simulink model "SensorFaultInj"  (R2013a)
settings: Solver=FixedStepDiscrete  SolverMode=SingleTasking  StartTime=0.0  StopTime=SimLength  FixedStep=SampleTime  RelTol=1e-3
values from neighbouring files (symbols this model uses):
  GlobalSeed = 10    [start_framework07.m]
  SampleTime = 0.01    [start_framework07.m]
  SimLength = 40    [start_framework07.m]
undefined symbols (not defined in the file or in its folder): DiscIntNeverNeededParam
libraries: dspswit3 x48, simulink x32
(part 9 of 9)

== system SensorFaultInj/FIM_Muster1/Parser Modul/parameter parser/Enabled Subsystem/param_fcn id 9/parser_fcn param id 2 ==
  input : Inport
  ex_sfun_paramfcn : S-Function  FunctionName=ex_sfun_paramfcn  EnableBusSupport=off  mask(Legacy Function){SFunctionSpec=double y1 = param_fcn(single u1, single u2, single u3), ShowSpec=on}
      mask prompts: ShowSpec "Display function specification"
      mask help:
      | This block allows you to call the legacy functions specified by the following Legacy Code Tool definition:
      | def.SFunctionName = 'ex_sfun_paramfcn';
      | def.OutputFcnSpec = 'double y1 = param_fcn(single u1, single u2, single u3)';
      | def.HeaderFiles = {'param_fcn.hpp'};
      | def.SourceFiles = {'param_fcn.cpp'};
      | def.Options.language = 'C++';
      mask Help: <p>This block was generated automatically by the Legacy Code Tool. For detailed help on this tool, call<a href="matlab:legacy_code('help')"> legacy_code('help')</a>.</p>
      mask Callback ShowSpec:
      | if strcmp(get_param(gcbh, 'ShowSpec'), 'on')
      |   set_param(gcbh, 'MaskDisplay', sprintf('fprintf(''%s'');', get_param(gcbh, 'SFunctionSpec')));
      | else
      |   set_param(gcbh, 'MaskDisplay', sprintf('fprintf(''%s'');', get_param(gcbh, 'FunctionName')));
      | end
      mask Display: fprintf('double y1 = param_fcn(single u1, single u2, single u3)');
  "fault_id " : Constant  Value=9  OutDataTypeStr=single
  "param_id " : Constant  Value=0  OutDataTypeStr=single
  output : Outport
  wires:
  "fault_id "/1 -> ex_sfun_paramfcn/1
  "param_id "/1 -> ex_sfun_paramfcn/2
  ex_sfun_paramfcn/1 -> output/1
  input/1 -> ex_sfun_paramfcn/3

== system SensorFaultInj/FIM_Muster1/Parser Modul/parameter parser/Enabled Subsystem/param_fcn id 9/parser_fcn param id 3 ==
  input : Inport
  ex_sfun_paramfcn : S-Function  FunctionName=ex_sfun_paramfcn  EnableBusSupport=off  mask(Legacy Function){SFunctionSpec=double y1 = param_fcn(single u1, single u2, single u3), ShowSpec=on}
      mask prompts: ShowSpec "Display function specification"
      mask help:
      | This block allows you to call the legacy functions specified by the following Legacy Code Tool definition:
      | def.SFunctionName = 'ex_sfun_paramfcn';
      | def.OutputFcnSpec = 'double y1 = param_fcn(single u1, single u2, single u3)';
      | def.HeaderFiles = {'param_fcn.hpp'};
      | def.SourceFiles = {'param_fcn.cpp'};
      | def.Options.language = 'C++';
      mask Help: <p>This block was generated automatically by the Legacy Code Tool. For detailed help on this tool, call<a href="matlab:legacy_code('help')"> legacy_code('help')</a>.</p>
      mask Callback ShowSpec:
      | if strcmp(get_param(gcbh, 'ShowSpec'), 'on')
      |   set_param(gcbh, 'MaskDisplay', sprintf('fprintf(''%s'');', get_param(gcbh, 'SFunctionSpec')));
      | else
      |   set_param(gcbh, 'MaskDisplay', sprintf('fprintf(''%s'');', get_param(gcbh, 'FunctionName')));
      | end
      mask Display: fprintf('double y1 = param_fcn(single u1, single u2, single u3)');
  "fault_id " : Constant  Value=9  OutDataTypeStr=single
  "param_id " : Constant  OutDataTypeStr=single
  output : Outport
  wires:
  "fault_id "/1 -> ex_sfun_paramfcn/1
  "param_id "/1 -> ex_sfun_paramfcn/2
  ex_sfun_paramfcn/1 -> output/1
  input/1 -> ex_sfun_paramfcn/3

== system SensorFaultInj/FIM_Muster2/Parser Modul/parameter parser/Enabled Subsystem/param_fcn id 0/parser_fcn param id 2 ==
  input : Inport
  ex_sfun_paramfcn : S-Function  FunctionName=ex_sfun_paramfcn  EnableBusSupport=off  mask(Legacy Function){SFunctionSpec=double y1 = param_fcn(single u1, single u2, single u3), ShowSpec=on}
      mask prompts: ShowSpec "Display function specification"
      mask help:
      | This block allows you to call the legacy functions specified by the following Legacy Code Tool definition:
      | def.SFunctionName = 'ex_sfun_paramfcn';
      | def.OutputFcnSpec = 'double y1 = param_fcn(single u1, single u2, single u3)';
      | def.HeaderFiles = {'param_fcn.hpp'};
      | def.SourceFiles = {'param_fcn.cpp'};
      | def.Options.language = 'C++';
      mask Help: <p>This block was generated automatically by the Legacy Code Tool. For detailed help on this tool, call<a href="matlab:legacy_code('help')"> legacy_code('help')</a>.</p>
      mask Callback ShowSpec:
      | if strcmp(get_param(gcbh, 'ShowSpec'), 'on')
      |   set_param(gcbh, 'MaskDisplay', sprintf('fprintf(''%s'');', get_param(gcbh, 'SFunctionSpec')));
      | else
      |   set_param(gcbh, 'MaskDisplay', sprintf('fprintf(''%s'');', get_param(gcbh, 'FunctionName')));
      | end
      mask Display: fprintf('double y1 = param_fcn(single u1, single u2, single u3)');
  "fault_id " : Constant  Value=0  OutDataTypeStr=single
  "param_id " : Constant  Value=0  OutDataTypeStr=single
  output : Outport
  wires:
  "fault_id "/1 -> ex_sfun_paramfcn/1
  "param_id "/1 -> ex_sfun_paramfcn/2
  ex_sfun_paramfcn/1 -> output/1
  input/1 -> ex_sfun_paramfcn/3

== system SensorFaultInj/FIM_Muster2/Parser Modul/parameter parser/Enabled Subsystem/param_fcn id 1/parser_fcn param id 2 ==
  input : Inport
  ex_sfun_paramfcn : S-Function  FunctionName=ex_sfun_paramfcn  EnableBusSupport=off  mask(Legacy Function){SFunctionSpec=double y1 = param_fcn(single u1, single u2, single u3), ShowSpec=on}
      mask prompts: ShowSpec "Display function specification"
      mask help:
      | This block allows you to call the legacy functions specified by the following Legacy Code Tool definition:
      | def.SFunctionName = 'ex_sfun_paramfcn';
      | def.OutputFcnSpec = 'double y1 = param_fcn(single u1, single u2, single u3)';
      | def.HeaderFiles = {'param_fcn.hpp'};
      | def.SourceFiles = {'param_fcn.cpp'};
      | def.Options.language = 'C++';
      mask Help: <p>This block was generated automatically by the Legacy Code Tool. For detailed help on this tool, call<a href="matlab:legacy_code('help')"> legacy_code('help')</a>.</p>
      mask Callback ShowSpec:
      | if strcmp(get_param(gcbh, 'ShowSpec'), 'on')
      |   set_param(gcbh, 'MaskDisplay', sprintf('fprintf(''%s'');', get_param(gcbh, 'SFunctionSpec')));
      | else
      |   set_param(gcbh, 'MaskDisplay', sprintf('fprintf(''%s'');', get_param(gcbh, 'FunctionName')));
      | end
      mask Display: fprintf('double y1 = param_fcn(single u1, single u2, single u3)');
  "fault_id " : Constant  OutDataTypeStr=single
  "param_id " : Constant  Value=0  OutDataTypeStr=single
  output : Outport
  wires:
  "fault_id "/1 -> ex_sfun_paramfcn/1
  "param_id "/1 -> ex_sfun_paramfcn/2
  ex_sfun_paramfcn/1 -> output/1
  input/1 -> ex_sfun_paramfcn/3

== system SensorFaultInj/FIM_Muster2/Parser Modul/parameter parser/Enabled Subsystem/param_fcn id 10/parser_fcn param id 0 ==
  input : Inport
  ex_sfun_paramfcn : S-Function  FunctionName=ex_sfun_paramfcn  EnableBusSupport=off  mask(Legacy Function){SFunctionSpec=double y1 = param_fcn(single u1, single u2, single u3), ShowSpec=on}
      mask prompts: ShowSpec "Display function specification"
      mask help:
      | This block allows you to call the legacy functions specified by the following Legacy Code Tool definition:
      | def.SFunctionName = 'ex_sfun_paramfcn';
      | def.OutputFcnSpec = 'double y1 = param_fcn(single u1, single u2, single u3)';
      | def.HeaderFiles = {'param_fcn.hpp'};
      | def.SourceFiles = {'param_fcn.cpp'};
      | def.Options.language = 'C++';
      mask Help: <p>This block was generated automatically by the Legacy Code Tool. For detailed help on this tool, call<a href="matlab:legacy_code('help')"> legacy_code('help')</a>.</p>
      mask Callback ShowSpec:
      | if strcmp(get_param(gcbh, 'ShowSpec'), 'on')
      |   set_param(gcbh, 'MaskDisplay', sprintf('fprintf(''%s'');', get_param(gcbh, 'SFunctionSpec')));
      | else
      |   set_param(gcbh, 'MaskDisplay', sprintf('fprintf(''%s'');', get_param(gcbh, 'FunctionName')));
      | end
      mask Display: fprintf('double y1 = param_fcn(single u1, single u2, single u3)');
  "fault_id " : Constant  Value=10  OutDataTypeStr=single
  "param_id " : Constant  Value=0  OutDataTypeStr=single
  output : Outport
  wires:
  "fault_id "/1 -> ex_sfun_paramfcn/1
  "param_id "/1 -> ex_sfun_paramfcn/2
  ex_sfun_paramfcn/1 -> output/1
  input/1 -> ex_sfun_paramfcn/3

== system SensorFaultInj/FIM_Muster2/Parser Modul/parameter parser/Enabled Subsystem/param_fcn id 10/parser_fcn param id 1 ==
  input : Inport
  ex_sfun_paramfcn : S-Function  FunctionName=ex_sfun_paramfcn  EnableBusSupport=off  mask(Legacy Function){SFunctionSpec=double y1 = param_fcn(single u1, single u2, single u3), ShowSpec=on}
      mask prompts: ShowSpec "Display function specification"
      mask help:
      | This block allows you to call the legacy functions specified by the following Legacy Code Tool definition:
      | def.SFunctionName = 'ex_sfun_paramfcn';
      | def.OutputFcnSpec = 'double y1 = param_fcn(single u1, single u2, single u3)';
      | def.HeaderFiles = {'param_fcn.hpp'};
      | def.SourceFiles = {'param_fcn.cpp'};
      | def.Options.language = 'C++';
      mask Help: <p>This block was generated automatically by the Legacy Code Tool. For detailed help on this tool, call<a href="matlab:legacy_code('help')"> legacy_code('help')</a>.</p>
      mask Callback ShowSpec:
      | if strcmp(get_param(gcbh, 'ShowSpec'), 'on')
      |   set_param(gcbh, 'MaskDisplay', sprintf('fprintf(''%s'');', get_param(gcbh, 'SFunctionSpec')));
      | else
      |   set_param(gcbh, 'MaskDisplay', sprintf('fprintf(''%s'');', get_param(gcbh, 'FunctionName')));
      | end
      mask Display: fprintf('double y1 = param_fcn(single u1, single u2, single u3)');
  "fault_id " : Constant  Value=10  OutDataTypeStr=single
  "param_id " : Constant  OutDataTypeStr=single
  output : Outport
  wires:
  "fault_id "/1 -> ex_sfun_paramfcn/1
  "param_id "/1 -> ex_sfun_paramfcn/2
  ex_sfun_paramfcn/1 -> output/1
  input/1 -> ex_sfun_paramfcn/3

== system SensorFaultInj/FIM_Muster2/Parser Modul/parameter parser/Enabled Subsystem/param_fcn id 11/parser_fcn param id 2 ==
  input : Inport
  ex_sfun_paramfcn : S-Function  FunctionName=ex_sfun_paramfcn  EnableBusSupport=off  mask(Legacy Function){SFunctionSpec=double y1 = param_fcn(single u1, single u2, single u3), ShowSpec=on}
      mask prompts: ShowSpec "Display function specification"
      mask help:
      | This block allows you to call the legacy functions specified by the following Legacy Code Tool definition:
      | def.SFunctionName = 'ex_sfun_paramfcn';
      | def.OutputFcnSpec = 'double y1 = param_fcn(single u1, single u2, single u3)';
      | def.HeaderFiles = {'param_fcn.hpp'};
      | def.SourceFiles = {'param_fcn.cpp'};
      | def.Options.language = 'C++';
      mask Help: <p>This block was generated automatically by the Legacy Code Tool. For detailed help on this tool, call<a href="matlab:legacy_code('help')"> legacy_code('help')</a>.</p>
      mask Callback ShowSpec:
      | if strcmp(get_param(gcbh, 'ShowSpec'), 'on')
      |   set_param(gcbh, 'MaskDisplay', sprintf('fprintf(''%s'');', get_param(gcbh, 'SFunctionSpec')));
      | else
      |   set_param(gcbh, 'MaskDisplay', sprintf('fprintf(''%s'');', get_param(gcbh, 'FunctionName')));
      | end
      mask Display: fprintf('double y1 = param_fcn(single u1, single u2, single u3)');
  "fault_id " : Constant  Value=11  OutDataTypeStr=single
  "param_id " : Constant  Value=0  OutDataTypeStr=single
  output : Outport
  wires:
  "fault_id "/1 -> ex_sfun_paramfcn/1
  "param_id "/1 -> ex_sfun_paramfcn/2
  ex_sfun_paramfcn/1 -> output/1
  input/1 -> ex_sfun_paramfcn/3

== system SensorFaultInj/FIM_Muster2/Parser Modul/parameter parser/Enabled Subsystem/param_fcn id 12/parser_fcn param id 2 ==
  input : Inport
  ex_sfun_paramfcn : S-Function  FunctionName=ex_sfun_paramfcn  EnableBusSupport=off  mask(Legacy Function){SFunctionSpec=double y1 = param_fcn(single u1, single u2, single u3), ShowSpec=on}
      mask prompts: ShowSpec "Display function specification"
      mask help:
      | This block allows you to call the legacy functions specified by the following Legacy Code Tool definition:
      | def.SFunctionName = 'ex_sfun_paramfcn';
      | def.OutputFcnSpec = 'double y1 = param_fcn(single u1, single u2, single u3)';
      | def.HeaderFiles = {'param_fcn.hpp'};
      | def.SourceFiles = {'param_fcn.cpp'};
      | def.Options.language = 'C++';
      mask Help: <p>This block was generated automatically by the Legacy Code Tool. For detailed help on this tool, call<a href="matlab:legacy_code('help')"> legacy_code('help')</a>.</p>
      mask Callback ShowSpec:
      | if strcmp(get_param(gcbh, 'ShowSpec'), 'on')
      |   set_param(gcbh, 'MaskDisplay', sprintf('fprintf(''%s'');', get_param(gcbh, 'SFunctionSpec')));
      | else
      |   set_param(gcbh, 'MaskDisplay', sprintf('fprintf(''%s'');', get_param(gcbh, 'FunctionName')));
      | end
      mask Display: fprintf('double y1 = param_fcn(single u1, single u2, single u3)');
  "fault_id " : Constant  Value=12  OutDataTypeStr=single
  "param_id " : Constant  Value=0  OutDataTypeStr=single
  output : Outport
  wires:
  "fault_id "/1 -> ex_sfun_paramfcn/1
  "param_id "/1 -> ex_sfun_paramfcn/2
  ex_sfun_paramfcn/1 -> output/1
  input/1 -> ex_sfun_paramfcn/3

== system SensorFaultInj/FIM_Muster2/Parser Modul/parameter parser/Enabled Subsystem/param_fcn id 2/parser_fcn param id 3 ==
  input : Inport
  ex_sfun_paramfcn : S-Function  FunctionName=ex_sfun_paramfcn  EnableBusSupport=off  mask(Legacy Function){SFunctionSpec=double y1 = param_fcn(single u1, single u2, single u3), ShowSpec=on}
      mask prompts: ShowSpec "Display function specification"
      mask help:
      | This block allows you to call the legacy functions specified by the following Legacy Code Tool definition:
      | def.SFunctionName = 'ex_sfun_paramfcn';
      | def.OutputFcnSpec = 'double y1 = param_fcn(single u1, single u2, single u3)';
      | def.HeaderFiles = {'param_fcn.hpp'};
      | def.SourceFiles = {'param_fcn.cpp'};
      | def.Options.language = 'C++';
      mask Help: <p>This block was generated automatically by the Legacy Code Tool. For detailed help on this tool, call<a href="matlab:legacy_code('help')"> legacy_code('help')</a>.</p>
      mask Callback ShowSpec:
      | if strcmp(get_param(gcbh, 'ShowSpec'), 'on')
      |   set_param(gcbh, 'MaskDisplay', sprintf('fprintf(''%s'');', get_param(gcbh, 'SFunctionSpec')));
      | else
      |   set_param(gcbh, 'MaskDisplay', sprintf('fprintf(''%s'');', get_param(gcbh, 'FunctionName')));
      | end
      mask Display: fprintf('double y1 = param_fcn(single u1, single u2, single u3)');
  "fault_id " : Constant  Value=2  OutDataTypeStr=single
  "param_id " : Constant  Value=0  OutDataTypeStr=single
  output : Outport
  wires:
  "fault_id "/1 -> ex_sfun_paramfcn/1
  "param_id "/1 -> ex_sfun_paramfcn/2
  ex_sfun_paramfcn/1 -> output/1
  input/1 -> ex_sfun_paramfcn/3

== system SensorFaultInj/FIM_Muster2/Parser Modul/parameter parser/Enabled Subsystem/param_fcn id 3/parser_fcn param id 2 ==
  input : Inport
  ex_sfun_paramfcn : S-Function  FunctionName=ex_sfun_paramfcn  EnableBusSupport=off  mask(Legacy Function){SFunctionSpec=double y1 = param_fcn(single u1, single u2, single u3), ShowSpec=on}
      mask prompts: ShowSpec "Display function specification"
      mask help:
      | This block allows you to call the legacy functions specified by the following Legacy Code Tool definition:
      | def.SFunctionName = 'ex_sfun_paramfcn';
      | def.OutputFcnSpec = 'double y1 = param_fcn(single u1, single u2, single u3)';
      | def.HeaderFiles = {'param_fcn.hpp'};
      | def.SourceFiles = {'param_fcn.cpp'};
      | def.Options.language = 'C++';
      mask Help: <p>This block was generated automatically by the Legacy Code Tool. For detailed help on this tool, call<a href="matlab:legacy_code('help')"> legacy_code('help')</a>.</p>
      mask Callback ShowSpec:
      | if strcmp(get_param(gcbh, 'ShowSpec'), 'on')
      |   set_param(gcbh, 'MaskDisplay', sprintf('fprintf(''%s'');', get_param(gcbh, 'SFunctionSpec')));
      | else
      |   set_param(gcbh, 'MaskDisplay', sprintf('fprintf(''%s'');', get_param(gcbh, 'FunctionName')));
      | end
      mask Display: fprintf('double y1 = param_fcn(single u1, single u2, single u3)');
  "fault_id " : Constant  Value=3  OutDataTypeStr=single
  "param_id " : Constant  Value=0  OutDataTypeStr=single
  output : Outport
  wires:
  "fault_id "/1 -> ex_sfun_paramfcn/1
  "param_id "/1 -> ex_sfun_paramfcn/2
  ex_sfun_paramfcn/1 -> output/1
  input/1 -> ex_sfun_paramfcn/3

== system SensorFaultInj/FIM_Muster2/Parser Modul/parameter parser/Enabled Subsystem/param_fcn id 4/parser_fcn param id 2 ==
  input : Inport
  ex_sfun_paramfcn : S-Function  FunctionName=ex_sfun_paramfcn  EnableBusSupport=off  mask(Legacy Function){SFunctionSpec=double y1 = param_fcn(single u1, single u2, single u3), ShowSpec=on}
      mask prompts: ShowSpec "Display function specification"
      mask help:
      | This block allows you to call the legacy functions specified by the following Legacy Code Tool definition:
      | def.SFunctionName = 'ex_sfun_paramfcn';
      | def.OutputFcnSpec = 'double y1 = param_fcn(single u1, single u2, single u3)';
      | def.HeaderFiles = {'param_fcn.hpp'};
      | def.SourceFiles = {'param_fcn.cpp'};
      | def.Options.language = 'C++';
      mask Help: <p>This block was generated automatically by the Legacy Code Tool. For detailed help on this tool, call<a href="matlab:legacy_code('help')"> legacy_code('help')</a>.</p>
      mask Callback ShowSpec:
      | if strcmp(get_param(gcbh, 'ShowSpec'), 'on')
      |   set_param(gcbh, 'MaskDisplay', sprintf('fprintf(''%s'');', get_param(gcbh, 'SFunctionSpec')));
      | else
      |   set_param(gcbh, 'MaskDisplay', sprintf('fprintf(''%s'');', get_param(gcbh, 'FunctionName')));
      | end
      mask Display: fprintf('double y1 = param_fcn(single u1, single u2, single u3)');
  "fault_id " : Constant  Value=4  OutDataTypeStr=single
  "param_id " : Constant  Value=0  OutDataTypeStr=single
  output : Outport
  wires:
  "fault_id "/1 -> ex_sfun_paramfcn/1
  "param_id "/1 -> ex_sfun_paramfcn/2
  ex_sfun_paramfcn/1 -> output/1
  input/1 -> ex_sfun_paramfcn/3

== system SensorFaultInj/FIM_Muster2/Parser Modul/parameter parser/Enabled Subsystem/param_fcn id 5/parser_fcn param id 2 ==
  input : Inport
  ex_sfun_paramfcn : S-Function  FunctionName=ex_sfun_paramfcn  EnableBusSupport=off  mask(Legacy Function){SFunctionSpec=double y1 = param_fcn(single u1, single u2, single u3), ShowSpec=on}
      mask prompts: ShowSpec "Display function specification"
      mask help:
      | This block allows you to call the legacy functions specified by the following Legacy Code Tool definition:
      | def.SFunctionName = 'ex_sfun_paramfcn';
      | def.OutputFcnSpec = 'double y1 = param_fcn(single u1, single u2, single u3)';
      | def.HeaderFiles = {'param_fcn.hpp'};
      | def.SourceFiles = {'param_fcn.cpp'};
      | def.Options.language = 'C++';
      mask Help: <p>This block was generated automatically by the Legacy Code Tool. For detailed help on this tool, call<a href="matlab:legacy_code('help')"> legacy_code('help')</a>.</p>
      mask Callback ShowSpec:
      | if strcmp(get_param(gcbh, 'ShowSpec'), 'on')
      |   set_param(gcbh, 'MaskDisplay', sprintf('fprintf(''%s'');', get_param(gcbh, 'SFunctionSpec')));
      | else
      |   set_param(gcbh, 'MaskDisplay', sprintf('fprintf(''%s'');', get_param(gcbh, 'FunctionName')));
      | end
      mask Display: fprintf('double y1 = param_fcn(single u1, single u2, single u3)');
  "fault_id " : Constant  Value=5  OutDataTypeStr=single
  "param_id " : Constant  Value=0  OutDataTypeStr=single
  output : Outport
  wires:
  "fault_id "/1 -> ex_sfun_paramfcn/1
  "param_id "/1 -> ex_sfun_paramfcn/2
  ex_sfun_paramfcn/1 -> output/1
  input/1 -> ex_sfun_paramfcn/3

== system SensorFaultInj/FIM_Muster2/Parser Modul/parameter parser/Enabled Subsystem/param_fcn id 6/parser_fcn param id 2 ==
  input : Inport
  ex_sfun_paramfcn : S-Function  FunctionName=ex_sfun_paramfcn  EnableBusSupport=off  mask(Legacy Function){SFunctionSpec=double y1 = param_fcn(single u1, single u2, single u3), ShowSpec=on}
      mask prompts: ShowSpec "Display function specification"
      mask help:
      | This block allows you to call the legacy functions specified by the following Legacy Code Tool definition:
      | def.SFunctionName = 'ex_sfun_paramfcn';
      | def.OutputFcnSpec = 'double y1 = param_fcn(single u1, single u2, single u3)';
      | def.HeaderFiles = {'param_fcn.hpp'};
      | def.SourceFiles = {'param_fcn.cpp'};
      | def.Options.language = 'C++';
      mask Help: <p>This block was generated automatically by the Legacy Code Tool. For detailed help on this tool, call<a href="matlab:legacy_code('help')"> legacy_code('help')</a>.</p>
      mask Callback ShowSpec:
      | if strcmp(get_param(gcbh, 'ShowSpec'), 'on')
      |   set_param(gcbh, 'MaskDisplay', sprintf('fprintf(''%s'');', get_param(gcbh, 'SFunctionSpec')));
      | else
      |   set_param(gcbh, 'MaskDisplay', sprintf('fprintf(''%s'');', get_param(gcbh, 'FunctionName')));
      | end
      mask Display: fprintf('double y1 = param_fcn(single u1, single u2, single u3)');
  "fault_id " : Constant  Value=6  OutDataTypeStr=single
  "param_id " : Constant  Value=0  OutDataTypeStr=single
  output : Outport
  wires:
  "fault_id "/1 -> ex_sfun_paramfcn/1
  "param_id "/1 -> ex_sfun_paramfcn/2
  ex_sfun_paramfcn/1 -> output/1
  input/1 -> ex_sfun_paramfcn/3

== system SensorFaultInj/FIM_Muster2/Parser Modul/parameter parser/Enabled Subsystem/param_fcn id 6/parser_fcn param id 3 ==
  input : Inport
  ex_sfun_paramfcn : S-Function  FunctionName=ex_sfun_paramfcn  EnableBusSupport=off  mask(Legacy Function){SFunctionSpec=double y1 = param_fcn(single u1, single u2, single u3), ShowSpec=on}
      mask prompts: ShowSpec "Display function specification"
      mask help:
      | This block allows you to call the legacy functions specified by the following Legacy Code Tool definition:
      | def.SFunctionName = 'ex_sfun_paramfcn';
      | def.OutputFcnSpec = 'double y1 = param_fcn(single u1, single u2, single u3)';
      | def.HeaderFiles = {'param_fcn.hpp'};
      | def.SourceFiles = {'param_fcn.cpp'};
      | def.Options.language = 'C++';
      mask Help: <p>This block was generated automatically by the Legacy Code Tool. For detailed help on this tool, call<a href="matlab:legacy_code('help')"> legacy_code('help')</a>.</p>
      mask Callback ShowSpec:
      | if strcmp(get_param(gcbh, 'ShowSpec'), 'on')
      |   set_param(gcbh, 'MaskDisplay', sprintf('fprintf(''%s'');', get_param(gcbh, 'SFunctionSpec')));
      | else
      |   set_param(gcbh, 'MaskDisplay', sprintf('fprintf(''%s'');', get_param(gcbh, 'FunctionName')));
      | end
      mask Display: fprintf('double y1 = param_fcn(single u1, single u2, single u3)');
  "fault_id " : Constant  Value=6  OutDataTypeStr=single
  "param_id " : Constant  OutDataTypeStr=single
  output : Outport
  wires:
  "fault_id "/1 -> ex_sfun_paramfcn/1
  "param_id "/1 -> ex_sfun_paramfcn/2
  ex_sfun_paramfcn/1 -> output/1
  input/1 -> ex_sfun_paramfcn/3

== system SensorFaultInj/FIM_Muster2/Parser Modul/parameter parser/Enabled Subsystem/param_fcn id 7/parser_fcn param id 0 ==
  input : Inport
  ex_sfun_paramfcn : S-Function  FunctionName=ex_sfun_paramfcn  EnableBusSupport=off  mask(Legacy Function){SFunctionSpec=double y1 = param_fcn(single u1, single u2, single u3), ShowSpec=on}
      mask prompts: ShowSpec "Display function specification"
      mask help:
      | This block allows you to call the legacy functions specified by the following Legacy Code Tool definition:
      | def.SFunctionName = 'ex_sfun_paramfcn';
      | def.OutputFcnSpec = 'double y1 = param_fcn(single u1, single u2, single u3)';
      | def.HeaderFiles = {'param_fcn.hpp'};
      | def.SourceFiles = {'param_fcn.cpp'};
      | def.Options.language = 'C++';
      mask Help: <p>This block was generated automatically by the Legacy Code Tool. For detailed help on this tool, call<a href="matlab:legacy_code('help')"> legacy_code('help')</a>.</p>
      mask Callback ShowSpec:
      | if strcmp(get_param(gcbh, 'ShowSpec'), 'on')
      |   set_param(gcbh, 'MaskDisplay', sprintf('fprintf(''%s'');', get_param(gcbh, 'SFunctionSpec')));
      | else
      |   set_param(gcbh, 'MaskDisplay', sprintf('fprintf(''%s'');', get_param(gcbh, 'FunctionName')));
      | end
      mask Display: fprintf('double y1 = param_fcn(single u1, single u2, single u3)');
  "fault_id " : Constant  Value=7  OutDataTypeStr=single
  "param_id " : Constant  Value=0  OutDataTypeStr=single
  output : Outport
  wires:
  "fault_id "/1 -> ex_sfun_paramfcn/1
  "param_id "/1 -> ex_sfun_paramfcn/2
  ex_sfun_paramfcn/1 -> output/1
  input/1 -> ex_sfun_paramfcn/3

== system SensorFaultInj/FIM_Muster2/Parser Modul/parameter parser/Enabled Subsystem/param_fcn id 7/parser_fcn param id 1 ==
  input : Inport
  ex_sfun_paramfcn : S-Function  FunctionName=ex_sfun_paramfcn  EnableBusSupport=off  mask(Legacy Function){SFunctionSpec=double y1 = param_fcn(single u1, single u2, single u3), ShowSpec=on}
      mask prompts: ShowSpec "Display function specification"
      mask help:
      | This block allows you to call the legacy functions specified by the following Legacy Code Tool definition:
      | def.SFunctionName = 'ex_sfun_paramfcn';
      | def.OutputFcnSpec = 'double y1 = param_fcn(single u1, single u2, single u3)';
      | def.HeaderFiles = {'param_fcn.hpp'};
      | def.SourceFiles = {'param_fcn.cpp'};
      | def.Options.language = 'C++';
      mask Help: <p>This block was generated automatically by the Legacy Code Tool. For detailed help on this tool, call<a href="matlab:legacy_code('help')"> legacy_code('help')</a>.</p>
      mask Callback ShowSpec:
      | if strcmp(get_param(gcbh, 'ShowSpec'), 'on')
      |   set_param(gcbh, 'MaskDisplay', sprintf('fprintf(''%s'');', get_param(gcbh, 'SFunctionSpec')));
      | else
      |   set_param(gcbh, 'MaskDisplay', sprintf('fprintf(''%s'');', get_param(gcbh, 'FunctionName')));
      | end
      mask Display: fprintf('double y1 = param_fcn(single u1, single u2, single u3)');
  "fault_id " : Constant  Value=7  OutDataTypeStr=single
  "param_id " : Constant  OutDataTypeStr=single
  output : Outport
  wires:
  "fault_id "/1 -> ex_sfun_paramfcn/1
  "param_id "/1 -> ex_sfun_paramfcn/2
  ex_sfun_paramfcn/1 -> output/1
  input/1 -> ex_sfun_paramfcn/3

== system SensorFaultInj/FIM_Muster2/Parser Modul/parameter parser/Enabled Subsystem/param_fcn id 8/parser_fcn param id 0 ==
  input : Inport
  ex_sfun_paramfcn : S-Function  FunctionName=ex_sfun_paramfcn  EnableBusSupport=off  mask(Legacy Function){SFunctionSpec=double y1 = param_fcn(single u1, single u2, single u3), ShowSpec=on}
      mask prompts: ShowSpec "Display function specification"
      mask help:
      | This block allows you to call the legacy functions specified by the following Legacy Code Tool definition:
      | def.SFunctionName = 'ex_sfun_paramfcn';
      | def.OutputFcnSpec = 'double y1 = param_fcn(single u1, single u2, single u3)';
      | def.HeaderFiles = {'param_fcn.hpp'};
      | def.SourceFiles = {'param_fcn.cpp'};
      | def.Options.language = 'C++';
      mask Help: <p>This block was generated automatically by the Legacy Code Tool. For detailed help on this tool, call<a href="matlab:legacy_code('help')"> legacy_code('help')</a>.</p>
      mask Callback ShowSpec:
      | if strcmp(get_param(gcbh, 'ShowSpec'), 'on')
      |   set_param(gcbh, 'MaskDisplay', sprintf('fprintf(''%s'');', get_param(gcbh, 'SFunctionSpec')));
      | else
      |   set_param(gcbh, 'MaskDisplay', sprintf('fprintf(''%s'');', get_param(gcbh, 'FunctionName')));
      | end
      mask Display: fprintf('double y1 = param_fcn(single u1, single u2, single u3)');
  "fault_id " : Constant  Value=8  OutDataTypeStr=single
  "param_id " : Constant  Value=0  OutDataTypeStr=single
  output : Outport
  wires:
  "fault_id "/1 -> ex_sfun_paramfcn/1
  "param_id "/1 -> ex_sfun_paramfcn/2
  ex_sfun_paramfcn/1 -> output/1
  input/1 -> ex_sfun_paramfcn/3

== system SensorFaultInj/FIM_Muster2/Parser Modul/parameter parser/Enabled Subsystem/param_fcn id 9/parser_fcn param id 1 ==
  input : Inport
  ex_sfun_paramfcn : S-Function  FunctionName=ex_sfun_paramfcn  EnableBusSupport=off  mask(Legacy Function){SFunctionSpec=double y1 = param_fcn(single u1, single u2, single u3), ShowSpec=on}
      mask prompts: ShowSpec "Display function specification"
      mask help:
      | This block allows you to call the legacy functions specified by the following Legacy Code Tool definition:
      | def.SFunctionName = 'ex_sfun_paramfcn';
      | def.OutputFcnSpec = 'double y1 = param_fcn(single u1, single u2, single u3)';
      | def.HeaderFiles = {'param_fcn.hpp'};
      | def.SourceFiles = {'param_fcn.cpp'};
      | def.Options.language = 'C++';
      mask Help: <p>This block was generated automatically by the Legacy Code Tool. For detailed help on this tool, call<a href="matlab:legacy_code('help')"> legacy_code('help')</a>.</p>
      mask Callback ShowSpec:
      | if strcmp(get_param(gcbh, 'ShowSpec'), 'on')
      |   set_param(gcbh, 'MaskDisplay', sprintf('fprintf(''%s'');', get_param(gcbh, 'SFunctionSpec')));
      | else
      |   set_param(gcbh, 'MaskDisplay', sprintf('fprintf(''%s'');', get_param(gcbh, 'FunctionName')));
      | end
      mask Display: fprintf('double y1 = param_fcn(single u1, single u2, single u3)');
  "fault_id " : Constant  Value=9  OutDataTypeStr=single
  "param_id " : Constant  Value=2  OutDataTypeStr=single
  output : Outport
  wires:
  "fault_id "/1 -> ex_sfun_paramfcn/1
  "param_id "/1 -> ex_sfun_paramfcn/2
  ex_sfun_paramfcn/1 -> output/1
  input/1 -> ex_sfun_paramfcn/3

== system SensorFaultInj/FIM_Muster2/Parser Modul/parameter parser/Enabled Subsystem/param_fcn id 9/parser_fcn param id 2 ==
  input : Inport
  ex_sfun_paramfcn : S-Function  FunctionName=ex_sfun_paramfcn  EnableBusSupport=off  mask(Legacy Function){SFunctionSpec=double y1 = param_fcn(single u1, single u2, single u3), ShowSpec=on}
      mask prompts: ShowSpec "Display function specification"
      mask help:
      | This block allows you to call the legacy functions specified by the following Legacy Code Tool definition:
      | def.SFunctionName = 'ex_sfun_paramfcn';
      | def.OutputFcnSpec = 'double y1 = param_fcn(single u1, single u2, single u3)';
      | def.HeaderFiles = {'param_fcn.hpp'};
      | def.SourceFiles = {'param_fcn.cpp'};
      | def.Options.language = 'C++';
      mask Help: <p>This block was generated automatically by the Legacy Code Tool. For detailed help on this tool, call<a href="matlab:legacy_code('help')"> legacy_code('help')</a>.</p>
      mask Callback ShowSpec:
      | if strcmp(get_param(gcbh, 'ShowSpec'), 'on')
      |   set_param(gcbh, 'MaskDisplay', sprintf('fprintf(''%s'');', get_param(gcbh, 'SFunctionSpec')));
      | else
      |   set_param(gcbh, 'MaskDisplay', sprintf('fprintf(''%s'');', get_param(gcbh, 'FunctionName')));
      | end
      mask Display: fprintf('double y1 = param_fcn(single u1, single u2, single u3)');
  "fault_id " : Constant  Value=9  OutDataTypeStr=single
  "param_id " : Constant  Value=0  OutDataTypeStr=single
  output : Outport
  wires:
  "fault_id "/1 -> ex_sfun_paramfcn/1
  "param_id "/1 -> ex_sfun_paramfcn/2
  ex_sfun_paramfcn/1 -> output/1
  input/1 -> ex_sfun_paramfcn/3

== system SensorFaultInj/FIM_Muster2/Parser Modul/parameter parser/Enabled Subsystem/param_fcn id 9/parser_fcn param id 3 ==
  input : Inport
  ex_sfun_paramfcn : S-Function  FunctionName=ex_sfun_paramfcn  EnableBusSupport=off  mask(Legacy Function){SFunctionSpec=double y1 = param_fcn(single u1, single u2, single u3), ShowSpec=on}
      mask prompts: ShowSpec "Display function specification"
      mask help:
      | This block allows you to call the legacy functions specified by the following Legacy Code Tool definition:
      | def.SFunctionName = 'ex_sfun_paramfcn';
      | def.OutputFcnSpec = 'double y1 = param_fcn(single u1, single u2, single u3)';
      | def.HeaderFiles = {'param_fcn.hpp'};
      | def.SourceFiles = {'param_fcn.cpp'};
      | def.Options.language = 'C++';
      mask Help: <p>This block was generated automatically by the Legacy Code Tool. For detailed help on this tool, call<a href="matlab:legacy_code('help')"> legacy_code('help')</a>.</p>
      mask Callback ShowSpec:
      | if strcmp(get_param(gcbh, 'ShowSpec'), 'on')
      |   set_param(gcbh, 'MaskDisplay', sprintf('fprintf(''%s'');', get_param(gcbh, 'SFunctionSpec')));
      | else
      |   set_param(gcbh, 'MaskDisplay', sprintf('fprintf(''%s'');', get_param(gcbh, 'FunctionName')));
      | end
      mask Display: fprintf('double y1 = param_fcn(single u1, single u2, single u3)');
  "fault_id " : Constant  Value=9  OutDataTypeStr=single
  "param_id " : Constant  OutDataTypeStr=single
  output : Outport
  wires:
  "fault_id "/1 -> ex_sfun_paramfcn/1
  "param_id "/1 -> ex_sfun_paramfcn/2
  ex_sfun_paramfcn/1 -> output/1
  input/1 -> ex_sfun_paramfcn/3
